simulink model "BC"  (R2019b)
settings: Solver=FixedStepDiscrete  StartTime=0.0  StopTime=stop_time  RelTol=1e-3
InitFcn:
  | sm_callback_init
StopFcn:
  | sm_callback_stop
values from neighbouring files (symbols this model uses):
  mp = sm_init_avalon_signals(mp)    [sm_callback_init.m]
libraries: simulink x5
settings Model: Creator=Ross  LastModifiedBy=bugsbunny
settings DataIOCC: ReturnWorkspaceOutputs=off
settings OptimizationCC: BlockReduction=off  ConditionallyExecuteInputs=off  DefaultParameterBehavior=Inlined
settings DebuggingCC: ReadBeforeWriteMsg=DisableAll  WriteAfterWriteMsg=DisableAll  WriteAfterReadMsg=DisableAll  AlgebraicLoopMsg=error  MultiTaskDSMMsg=none  SingleTaskRateTransMsg=error  PregeneratedLibrarySubsystemCodeDiagnostic=none  ArithmeticOperatorsInVariantConditions=warning
settings HardwareCC: ProdBitPerPointer=32  ProdBitPerSizeT=32  ProdBitPerPtrDiffT=32  ProdLargestAtomicFloat=None  ProdIntDivRoundTo=Undefined  ProdEndianess=Unspecified  ProdWordSize=32  ProdHWDeviceType=ASIC/FPGA->ASIC/FPGA  TargetBitPerPointer=64  TargetBitPerSizeT=64  TargetBitPerPtrDiffT=64  TargetLongLongMode=on  TargetIntDivRoundTo=Zero  TargetEndianess=LittleEndian  TargetWordSize=64  TargetHWDeviceType=Custom Processor->MATLAB Host Computer  ProdEqTarget=off
settings ModelReferenceCC: UpdateModelReferenceTargets=IfOutOfDate
settings SFSimCC: SFSimEcho=off  SimUseLocalCustomCode=off  CustomCodeUndefinedFunction=UseInterfaceOnly
settings RTWCC: RTWUseLocalCustomCode=off

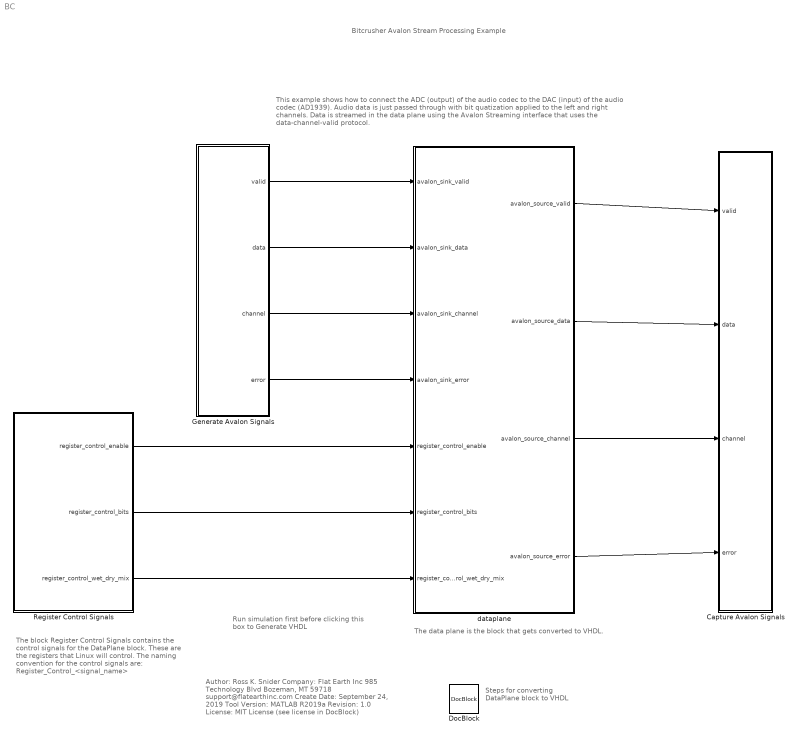
== system BC ==
  note: The data plane is the block that gets converted to VHDL.
  note: Author:          Ross K. Snider
      | Company:     Flat Earth Inc
      |                       985 Technology Blvd
      |                       Bozeman, MT 59718
      |                       support@flatearthinc.com
      | Create Date:  September 24, 2019
      | Tool Version:  MATLAB R2019a
      | Revision:        1.0
      | License:          MIT License (see license in DocBlock)
  note: This example shows how to connect the ADC (output) of the audio codec to the DAC (input) of the audio codec (AD1939). Audio data is just passed through with bit quatization applied to the left and right channels. Data is streamed in the data plane using the Avalon Streaming interface that uses the data-channel-valid protocol.
  note: Steps for converting
      | DataPlane block
      | to VHDL
  note: Bitcrusher
      | Avalon Stream Processing Example
  note: Run simulation first
      | before clicking this box to
      | Generate VHDL
  note: The block Register Control Signals contains
      | the control signals for the DataPlane block.
      | These are the registers that Linux will control.
      | The naming convention for the control
      | signals are:  Register_Control_<signal_name>
  Capture Avalon Signals : Subsystem
  DocBlock : simulink/Model-Wide Utilities/DocBlock  DocumentType=HTML
  Generate Avalon Signals : Subsystem
  Register Control Signals : Subsystem
  dataplane : Subsystem  TreatAsAtomicUnit=on
  wires:
  Generate Avalon Signals/2(data) -> dataplane/2(avalon_sink_data)
  Generate Avalon Signals/1(valid) -> dataplane/1(avalon_sink_valid)
  Generate Avalon Signals/3(channel) -> dataplane/3(avalon_sink_channel)
  Generate Avalon Signals/4(error) -> dataplane/4(avalon_sink_error)
  dataplane/2(avalon_source_data) -> Capture Avalon Signals/2(data)
  dataplane/1(avalon_source_valid) -> Capture Avalon Signals/1(valid)
  dataplane/3(avalon_source_channel) -> Capture Avalon Signals/3(channel)
  dataplane/4(avalon_source_error) -> Capture Avalon Signals/4(error)
  Register Control Signals/2(register_control_bits) -> dataplane/6(register_control_bits)
  Register Control Signals/1(register_control_enable) -> dataplane/5(register_control_enable)
  Register Control Signals/3(register_control_wet_dry_mix) -> dataplane/7(register_control_wet_dry_mix)

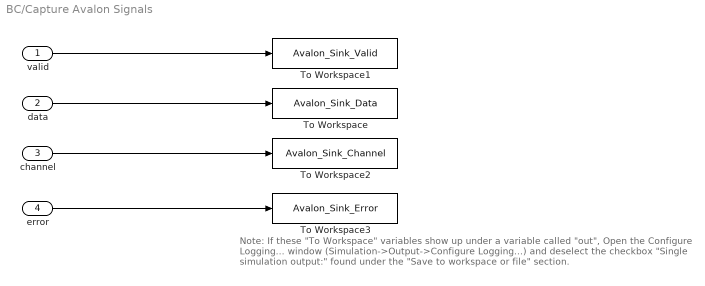
== system BC/Capture Avalon Signals ==
  note: Note:  If these "To Workspace" variables show up under a variable called "out",
      | Open the Configure Logging... window (Simulation->Output->Configure Logging...)
      | and deselect the checkbox "Single simulation output:" found under the "Save to workspace or file" section.
  valid : Inport
  data : Inport  Port=2
  channel : Inport  Port=3
  error : Inport  Port=4
  To Workspace : ToWorkspace  VariableName=Avalon_Sink_Data  SaveFormat=Timeseries  SampleTime=-1
  To Workspace1 : ToWorkspace  VariableName=Avalon_Sink_Valid  SaveFormat=Timeseries  SampleTime=-1
  To Workspace2 : ToWorkspace  VariableName=Avalon_Sink_Channel  SaveFormat=Timeseries  SampleTime=-1
  To Workspace3 : ToWorkspace  VariableName=Avalon_Sink_Error  SaveFormat=Timeseries  SampleTime=-1
  wires:
  data/1 -> To Workspace/1
  valid/1 -> To Workspace1/1
  error/1 -> To Workspace3/1
  channel/1 -> To Workspace2/1

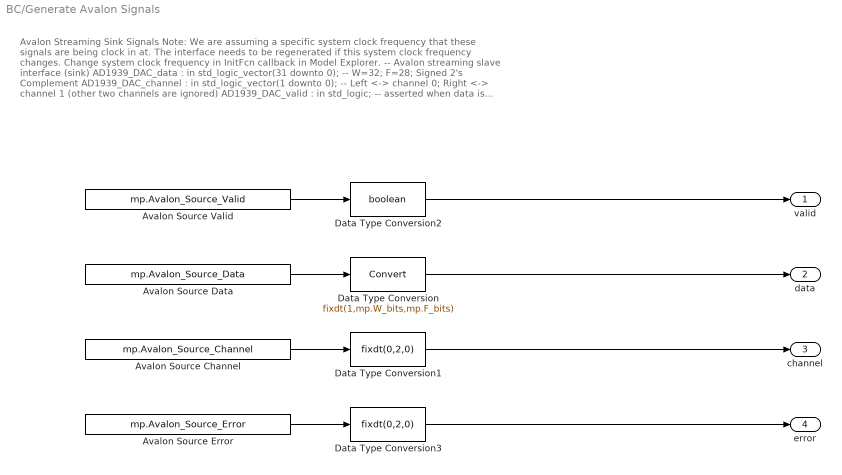
== system BC/Generate Avalon Signals ==
  note: Avalon Streaming Sink Signals
      | Note: We are assuming a specific system clock frequency that these signals are being clock in at.
      | The interface needs to be regenerated if this system clock frequency changes. Change system clock frequency in InitFcn callback in Model Explorer.
      |
      | -- Avalon streaming slave interface (sink)
      | AD1939_DAC_data : in std_logic_vector(31 downto 0); -- W=32; F=28; Signed 2's Complement
      | AD1939_DAC_channel : in std_logic_vector(1 downto 0); -- Left <-> channel 0; Right <-> channel 1 (other two channels are ignored)
      | AD1939_DAC_valid : in std_logic; -- asserted when data is valid
      | AD1939_DAC_error : in std_logic_vector(1 downto 0) -- error channel is ignored, assumed to be error free at this point
      |
      | For more information on the data-channel-valid protocol, s ee chapter 5 in Intel's Avalon Interfaced Specification (p. 40) at https://www.intel.com/content/dam/www/programmable/us/en/pdfs/literature/manual/mnl_avalon_spec.pdf
  Avalon Source Channel : FromWorkspace  VariableName=mp.Avalon_Source_Channel  OutDataTypeStr=double  SampleTime=mp.Ts_system
  "Avalon Source Data " : FromWorkspace  VariableName=mp.Avalon_Source_Data  OutDataTypeStr=double  SampleTime=mp.Ts_system
  Avalon Source Error : FromWorkspace  VariableName=mp.Avalon_Source_Error  OutDataTypeStr=double  SampleTime=mp.Ts_system
  Avalon Source Valid : FromWorkspace  VariableName=mp.Avalon_Source_Valid  OutDataTypeStr=double  SampleTime=mp.Ts_system
  Data Type Conversion : DataTypeConversion  OutDataTypeStr=fixdt(1,mp.W_bits,mp.F_bits)
  Data Type Conversion1 : DataTypeConversion  OutDataTypeStr=fixdt(0,2,0)
  Data Type Conversion2 : DataTypeConversion  OutDataTypeStr=boolean
  Data Type Conversion3 : DataTypeConversion  OutDataTypeStr=fixdt(0,2,0)
  valid : Outport  VectorParamsAs1DForOutWhenUnconnected=off
  data : Outport  Port=2  VectorParamsAs1DForOutWhenUnconnected=off
  channel : Outport  Port=3  VectorParamsAs1DForOutWhenUnconnected=off
  error : Outport  Port=4  VectorParamsAs1DForOutWhenUnconnected=off
  wires:
  Data Type Conversion1/1 -> channel/1
  Data Type Conversion2/1 -> valid/1
  Avalon Source Error/1 -> Data Type Conversion3/1
  Data Type Conversion/1 -> data/1
  Avalon Source Valid/1 -> Data Type Conversion2/1
  Data Type Conversion3/1 -> error/1
  Avalon Source Channel/1 -> Data Type Conversion1/1
  "Avalon Source Data "/1 -> Data Type Conversion/1

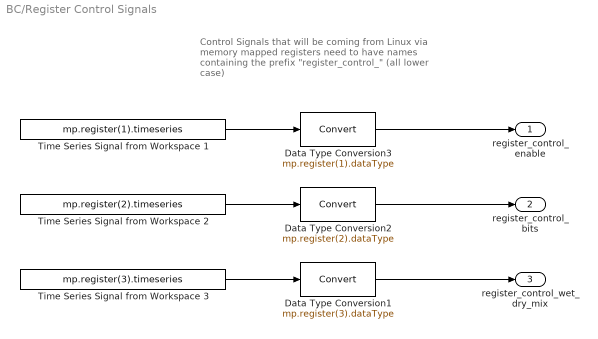
== system BC/Register Control Signals ==
  note: Control Signals that will be coming from Linux via
      | memory mapped registers need to have names
      | containing the prefix "register_control_"
      | (all lower case)
  Data Type Conversion1 : DataTypeConversion  OutDataTypeStr=mp.register(3).dataType
  Data Type Conversion2 : DataTypeConversion  OutDataTypeStr=mp.register(2).dataType
  Data Type Conversion3 : DataTypeConversion  OutDataTypeStr=mp.register(1).dataType
  Time Series Signal from Workspace 1 : FromWorkspace  VariableName=mp.register(1).timeseries  OutDataTypeStr=double  SampleTime=mp.Ts_system
  Time Series Signal from Workspace 2 : FromWorkspace  VariableName=mp.register(2).timeseries  OutDataTypeStr=double  SampleTime=mp.Ts_system
  Time Series Signal from Workspace 3 : FromWorkspace  VariableName=mp.register(3).timeseries  OutDataTypeStr=double  SampleTime=mp.Ts_system
  register_control_enable : Outport  VectorParamsAs1DForOutWhenUnconnected=off
  register_control_bits : Outport  Port=2  VectorParamsAs1DForOutWhenUnconnected=off
  register_control_wet_dry_mix : Outport  Port=3  VectorParamsAs1DForOutWhenUnconnected=off
  wires:
  Time Series Signal from Workspace 2/1 -> Data Type Conversion2/1
  Data Type Conversion2/1 -> register_control_bits/1
  Time Series Signal from Workspace 1/1 -> Data Type Conversion3/1
  Data Type Conversion3/1 -> register_control_enable/1
  Time Series Signal from Workspace 3/1 -> Data Type Conversion1/1
  Data Type Conversion1/1 -> register_control_wet_dry_mix/1

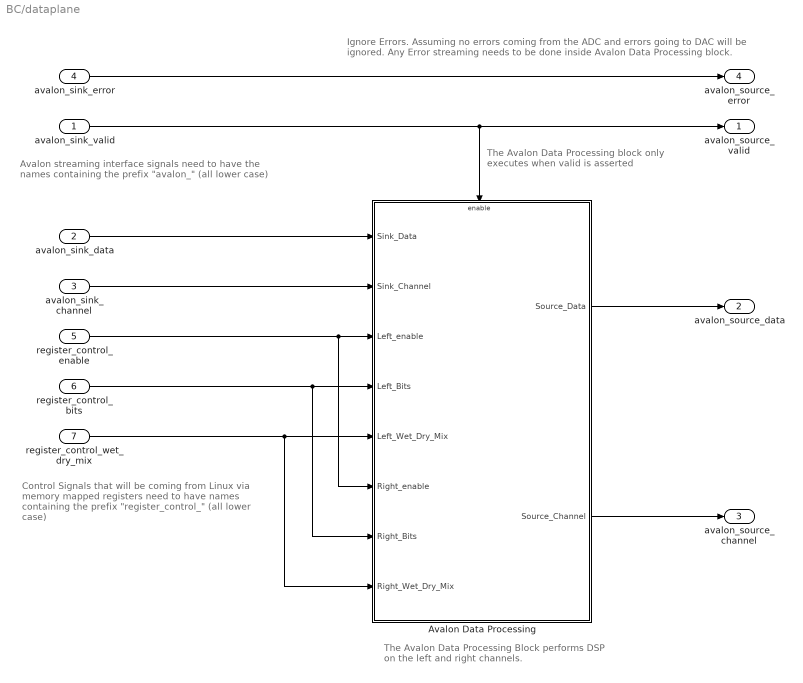
== system BC/dataplane ==
  note: Control Signals that will be coming from Linux via
      | memory mapped registers need to have names
      | containing the prefix "register_control_"
      | (all lower case)
  note: The Avalon Data Processing Block
      | performs DSP on the left and right channels.
  note: The Avalon Data Processing block
      | only executes when valid is asserted
  note: Ignore Errors.
      | Assuming no errors coming from the ADC and errors going to DAC will be ignored.
      | Any Error streaming needs to be done inside Avalon Data Processing block.
  note: Avalon streaming interface signals need to have the
      | names containing the prefix "avalon_"
      | (all lower case)
  avalon_sink_valid : Inport
  avalon_sink_data : Inport  Port=2
  avalon_sink_channel : Inport  Port=3
  avalon_sink_error : Inport  Port=4
  register_control_enable : Inport  Port=5
  register_control_bits : Inport  Port=6
  register_control_wet_dry_mix : Inport  Port=7
  Avalon Data Processing : Subsystem  TreatAsAtomicUnit=on
  avalon_source_valid : Outport  VectorParamsAs1DForOutWhenUnconnected=off
  avalon_source_data : Outport  Port=2  VectorParamsAs1DForOutWhenUnconnected=off
  avalon_source_channel : Outport  Port=3  VectorParamsAs1DForOutWhenUnconnected=off
  avalon_source_error : Outport  Port=4  VectorParamsAs1DForOutWhenUnconnected=off
  wires:
  avalon_sink_channel/1 -> Avalon Data Processing/2(Sink_Channel)
  avalon_sink_error/1 -> avalon_source_error/1
  Avalon Data Processing/1(Source_Data) -> avalon_source_data/1
  avalon_sink_valid/1 -> avalon_source_valid/1, Avalon Data Processing/Enable
  avalon_sink_data/1 -> Avalon Data Processing/1(Sink_Data)
  Avalon Data Processing/2(Source_Channel) -> avalon_source_channel/1
  register_control_bits/1 -> Avalon Data Processing/7(Right_Bits), Avalon Data Processing/4(Left_Bits)
  register_control_enable/1 -> Avalon Data Processing/6(Right_enable), Avalon Data Processing/3(Left_enable)
  register_control_wet_dry_mix/1 -> Avalon Data Processing/8(Right_Wet_Dry_Mix), Avalon Data Processing/5(Left_Wet_Dry_Mix)

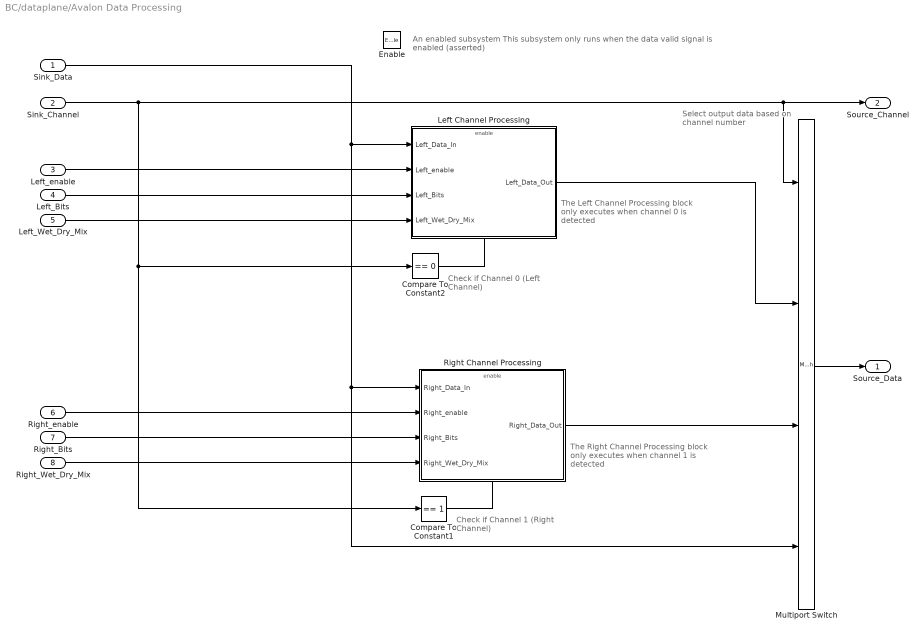
== system BC/dataplane/Avalon Data Processing ==
  note: Select output data
      | based on channel number
  note: Check if Channel 0
      | (Left Channel)
  note: The Left Channel Processing block
      | only executes when channel 0
      | is detected
  note: The Right Channel Processing block
      | only executes when channel 1
      | is detected
  note: Check if Channel 1
      | (Right Channel)
  note: An enabled subsystem
      | This subsystem only runs when the data valid signal is enabled (asserted)
  Sink_Data : Inport
  Sink_Channel : Inport  Port=2
  Left_enable : Inport  Port=3
  Left_Bits : Inport  Port=4
  Left_Wet_Dry_Mix : Inport  Port=5
  Right_enable : Inport  Port=6
  Right_Bits : Inport  Port=7
  Right_Wet_Dry_Mix : Inport  Port=8
  Enable : EnablePort
  Compare To Constant1 : simulink/Logic and Bit Operations/Compare To Constant  relop===  const=1  OutDataTypeStr=boolean
  Compare To Constant2 : simulink/Logic and Bit Operations/Compare To Constant  relop===  const=0  OutDataTypeStr=boolean
  Left Channel Processing : Subsystem  TreatAsAtomicUnit=on
  Multiport Switch : MultiPortSwitch  DataPortOrder=Zero-based contiguous  zeroidx=on
  Right Channel Processing : Subsystem  TreatAsAtomicUnit=on
  Source_Data : Outport  InitialOutput=0  VectorParamsAs1DForOutWhenUnconnected=off
  Source_Channel : Outport  Port=2  InitialOutput=0  VectorParamsAs1DForOutWhenUnconnected=off
  wires:
  Sink_Channel/1 -> Compare To Constant1/1, Compare To Constant2/1, Source_Channel/1, Multiport Switch/1
  Compare To Constant2/1 -> Left Channel Processing/Enable
  Compare To Constant1/1 -> Right Channel Processing/Enable
  Sink_Data/1 -> Multiport Switch/4, Right Channel Processing/1(Right_Data_In), Left Channel Processing/1(Left_Data_In)
  Left Channel Processing/1("Left_Data_Out ") -> Multiport Switch/2
  Right Channel Processing/1("Right_Data_Out ") -> Multiport Switch/3
  Multiport Switch/1 -> Source_Data/1
  Left_Bits/1 -> Left Channel Processing/3(Left_Bits)
  Right_Bits/1 -> Right Channel Processing/3(Right_Bits)
  Left_enable/1 -> Left Channel Processing/2(Left_enable)
  Right_enable/1 -> Right Channel Processing/2(Right_enable)
  Left_Wet_Dry_Mix/1 -> Left Channel Processing/4(Left_Wet_Dry_Mix)
  Right_Wet_Dry_Mix/1 -> Right Channel Processing/4(Right_Wet_Dry_Mix)

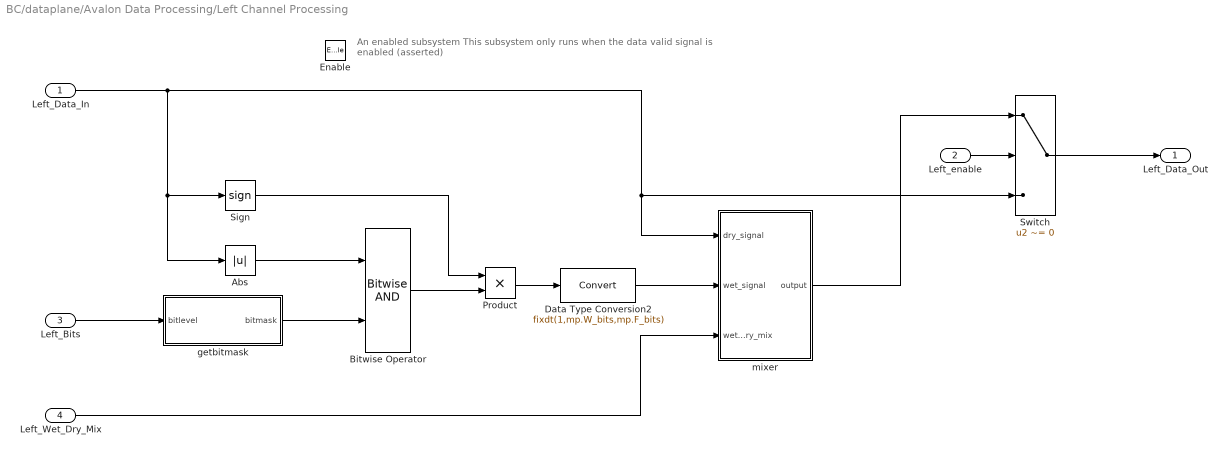
== system BC/dataplane/Avalon Data Processing/Left Channel Processing ==
  note: An enabled subsystem
      | This subsystem only runs when the data valid signal is enabled (asserted)
  Left_Data_In : Inport
  Left_enable : Inport  Port=2
  Left_Bits : Inport  Port=3
  Left_Wet_Dry_Mix : Inport  Port=4
  Enable : EnablePort
  Abs : Abs  OutDataTypeStr=fixdt(0,32,28)
  Bitwise Operator : simulink/Logic and Bit Operations/Bitwise Operator  logicop=AND  UseBitMask=off  NumInputPorts=2  BitMask=bin2dec('11011001')  BitMaskRealWorld=Stored Integer
  Data Type Conversion2 : DataTypeConversion  OutDataTypeStr=fixdt(1,mp.W_bits,mp.F_bits)
  Product : Product
  Sign : Signum
  Switch : Switch  Criteria=u2 ~= 0
  getbitmask : MATLAB Function  TreatAsAtomicUnit=on
  mixer : Subsystem
  "Left_Data_Out " : Outport  InitialOutput=0  VectorParamsAs1DForOutWhenUnconnected=off
  wires:
  Left_Bits/1 -> getbitmask/1(bitlevel)
  getbitmask/1(bitmask) -> Bitwise Operator/2
  Left_Data_In/1 -> Abs/1, Sign/1, mixer/1(dry_signal), Switch/3
  Abs/1 -> Bitwise Operator/1
  Product/1 -> Data Type Conversion2/1
  Bitwise Operator/1 -> Product/2
  Sign/1 -> Product/1
  Switch/1 -> "Left_Data_Out "/1
  Data Type Conversion2/1 -> mixer/2(wet_signal)
  Left_Wet_Dry_Mix/1 -> mixer/3(wet_dry_mix)
  Left_enable/1 -> Switch/2
  mixer/1(output) -> Switch/1

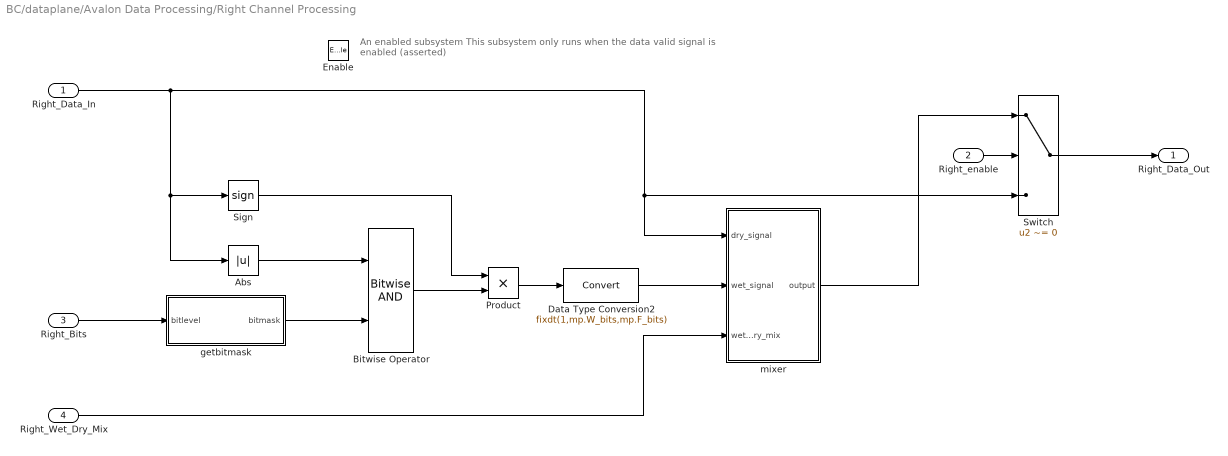
== system BC/dataplane/Avalon Data Processing/Right Channel Processing ==
  note: An enabled subsystem
      | This subsystem only runs when the data valid signal is enabled (asserted)
  Right_Data_In : Inport
  Right_enable : Inport  Port=2
  Right_Bits : Inport  Port=3
  Right_Wet_Dry_Mix : Inport  Port=4
  Enable : EnablePort
  Abs : Abs  OutDataTypeStr=fixdt(0,32,28)
  Bitwise Operator : simulink/Logic and Bit Operations/Bitwise Operator  logicop=AND  UseBitMask=off  NumInputPorts=2  BitMask=bin2dec('11011001')  BitMaskRealWorld=Stored Integer
  Data Type Conversion2 : DataTypeConversion  OutDataTypeStr=fixdt(1,mp.W_bits,mp.F_bits)
  Product : Product
  Sign : Signum
  Switch : Switch  Criteria=u2 ~= 0
  getbitmask : MATLAB Function  TreatAsAtomicUnit=on
  mixer : Subsystem
  "Right_Data_Out " : Outport  InitialOutput=0  VectorParamsAs1DForOutWhenUnconnected=off
  wires:
  Right_Bits/1 -> getbitmask/1(bitlevel)
  getbitmask/1(bitmask) -> Bitwise Operator/2
  Right_Data_In/1 -> Abs/1, Sign/1, Switch/3, mixer/1(dry_signal)
  Abs/1 -> Bitwise Operator/1
  Product/1 -> Data Type Conversion2/1
  Bitwise Operator/1 -> Product/2
  Sign/1 -> Product/1
  Switch/1 -> "Right_Data_Out "/1
  Data Type Conversion2/1 -> mixer/2(wet_signal)
  Right_Wet_Dry_Mix/1 -> mixer/3(wet_dry_mix)
  mixer/1(output) -> Switch/1
  Right_enable/1 -> Switch/2

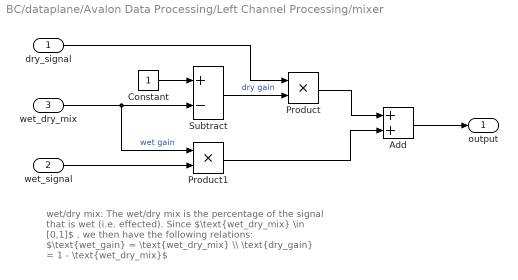
== system BC/dataplane/Avalon Data Processing/Left Channel Processing/mixer ==
  note: wet/dry mix:
      | The wet/dry mix is the percentage of the signal that is wet (i.e. effected).
      |
      | Since $\text{wet_dry_mix} \in [0,1]$ , we then have the following relations:
      | $\text{wet_gain} = \text{wet_dry_mix} \\ \text{dry_gain} = 1 - \text{wet_dry_mix}$
  dry_signal : Inport
  wet_signal : Inport  Port=2
  wet_dry_mix : Inport  Port=3
  Add : Sum  OutDataTypeStr=fixdt(1,mp.W_bits,mp.F_bits)
  Constant : Constant  OutDataTypeStr=Inherit: Inherit via back propagation  SampleTime=-1
  Product : Product  OutDataTypeStr=Inherit: Keep MSB
  Product1 : Product  OutDataTypeStr=Inherit: Keep MSB
  Subtract : Sum  Inputs=+-  InputSameDT=on  OutDataTypeStr=Inherit: Same as first input
  output : Outport  VectorParamsAs1DForOutWhenUnconnected=off
  wires:
  Add/1 -> output/1
  Constant/1 -> Subtract/1
  wet_dry_mix/1 -> Product1/1, Subtract/2  "wet gain"
  Product/1 -> Add/1
  Product1/1 -> Add/2
  wet_signal/1 -> Product1/2
  dry_signal/1 -> Product/1
  Subtract/1 -> Product/2  "dry gain"

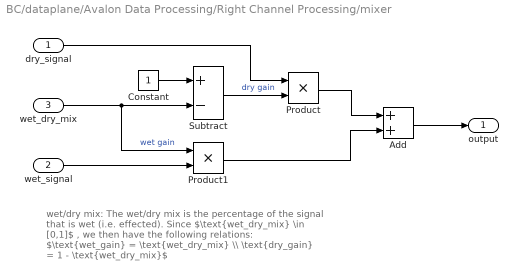
== system BC/dataplane/Avalon Data Processing/Right Channel Processing/mixer ==
  note: wet/dry mix:
      | The wet/dry mix is the percentage of the signal that is wet (i.e. effected).
      |
      | Since $\text{wet_dry_mix} \in [0,1]$ , we then have the following relations:
      | $\text{wet_gain} = \text{wet_dry_mix} \\ \text{dry_gain} = 1 - \text{wet_dry_mix}$
  dry_signal : Inport
  wet_signal : Inport  Port=2
  wet_dry_mix : Inport  Port=3
  Add : Sum  OutDataTypeStr=fixdt(1,mp.W_bits,mp.F_bits)
  Constant : Constant  OutDataTypeStr=Inherit: Inherit via back propagation  SampleTime=-1
  Product : Product  OutDataTypeStr=Inherit: Keep MSB
  Product1 : Product  OutDataTypeStr=Inherit: Keep MSB
  Subtract : Sum  Inputs=+-  InputSameDT=on  OutDataTypeStr=Inherit: Same as first input
  output : Outport  VectorParamsAs1DForOutWhenUnconnected=off
  wires:
  Product1/1 -> Add/2
  Product/1 -> Add/1
  dry_signal/1 -> Product/1
  Subtract/1 -> Product/2  "dry gain"
  wet_dry_mix/1 -> Product1/1, Subtract/2  "wet gain"
  Constant/1 -> Subtract/1
  Add/1 -> output/1
  wet_signal/1 -> Product1/2

== matlab function BC/dataplane/Avalon Data Processing/Right Channel Processing/getbitmask ==
  data: bitlevel input; bitmask output
function bitmask = getbitmask(bitlevel)
bitmask=fi(0,0,32,28);
switch(bitlevel)
    case 0
        bitmask = fi(0.0000000000000000000000000000,0,32,28);
    case 1
        bitmask = fi(8.0000000000000000000000000000,0,32,28);
    case 2
        bitmask = fi(12.0000000000000000000000000000,0,32,28);
    case 3
        bitmask = fi(14.0000000000000000000000000000,0,32,28);
    case 4
        bitmask = fi(15.0000000000000000000000000000,0,32,28);
    case 5
        bitmask = fi(15.5000000000000000000000000000,0,32,28);
    case 6
        bitmask = fi(15.7500000000000000000000000000,0,32,28);
    case 7
        bitmask = fi(15.8750000000000000000000000000,0,32,28);
    case 8
        bitmask = fi(15.9375000000000000000000000000,0,32,28);
    case 9
        bitmask = fi(15.9687500000000000000000000000,0,32,28);
    case 10
        bitmask = fi(15.9843750000000000000000000000,0,32,28);
    case 11
        bitmask = fi(15.9921875000000000000000000000,0,32,28);
    case 12
        bitmask = fi(15.9960937500000000000000000000,0,32,28);
    case 13
        bitmask = fi(15.9980468750000000000000000000,0,32,28);
    case 14
        bitmask = fi(15.9990234375000000000000000000,0,32,28);
    case 15
        bitmask = fi(15.9995117187500000000000000000,0,32,28);
    case 16
        bitmask = fi(15.9997558593750000000000000000,0,32,28);
    case 17
        bitmask = fi(15.9998779296875000000000000000,0,32,28);
    case 18
        bitmask = fi(15.9999389648437500000000000000,0,32,28);
    case 19
        bitmask = fi(15.9999694824218750000000000000,0,32,28);
    case 20
        bitmask = fi(15.9999847412109375000000000000,0,32,28);
    case 21
        bitmask = fi(15.9999923706054687500000000000,0,32,28);
    case 22
        bitmask = fi(15.9999961853027343750000000000,0,32,28);
    case 23
        bitmask = fi(15.9999980926513671875000000000,0,32,28);
    case 24
        bitmask = fi(15.9999990463256835937500000000,0,32,28);
    case 25
        bitmask = fi(15.9999995231628417968750000000,0,32,28);
    case 26
        bitmask = fi(15.9999997615814208984375000000,0,32,28);
    case 27
        bitmask = fi(15.9999998807907104492187500000,0,32,28);
    case 28
        bitmask = fi(15.9999999403953552246093750000,0,32,28);
    case 29
        bitmask = fi(15.9999999701976776123046875000,0,32,28);
    case 30
        bitmask = fi(15.9999999850988388061523437500,0,32,28);
    case 31
        bitmask = fi(15.9999999925494194030761718750,0,32,28);
    case 32
        bitmask = fi(15.9999999962747097015380859375,0,32,28);
end

== matlab function BC/dataplane/Avalon Data Processing/Left Channel Processing/getbitmask ==
  data: bitlevel input; bitmask output
function bitmask = getbitmask(bitlevel)
bitmask=fi(0,0,32,28);
switch(bitlevel)
    case 0
        bitmask = fi(0.0000000000000000000000000000,0,32,28);
    case 1
        bitmask = fi(8.0000000000000000000000000000,0,32,28);
    case 2
        bitmask = fi(12.0000000000000000000000000000,0,32,28);
    case 3
        bitmask = fi(14.0000000000000000000000000000,0,32,28);
    case 4
        bitmask = fi(15.0000000000000000000000000000,0,32,28);
    case 5
        bitmask = fi(15.5000000000000000000000000000,0,32,28);
    case 6
        bitmask = fi(15.7500000000000000000000000000,0,32,28);
    case 7
        bitmask = fi(15.8750000000000000000000000000,0,32,28);
    case 8
        bitmask = fi(15.9375000000000000000000000000,0,32,28);
    case 9
        bitmask = fi(15.9687500000000000000000000000,0,32,28);
    case 10
        bitmask = fi(15.9843750000000000000000000000,0,32,28);
    case 11
        bitmask = fi(15.9921875000000000000000000000,0,32,28);
    case 12
        bitmask = fi(15.9960937500000000000000000000,0,32,28);
    case 13
        bitmask = fi(15.9980468750000000000000000000,0,32,28);
    case 14
        bitmask = fi(15.9990234375000000000000000000,0,32,28);
    case 15
        bitmask = fi(15.9995117187500000000000000000,0,32,28);
    case 16
        bitmask = fi(15.9997558593750000000000000000,0,32,28);
    case 17
        bitmask = fi(15.9998779296875000000000000000,0,32,28);
    case 18
        bitmask = fi(15.9999389648437500000000000000,0,32,28);
    case 19
        bitmask = fi(15.9999694824218750000000000000,0,32,28);
    case 20
        bitmask = fi(15.9999847412109375000000000000,0,32,28);
    case 21
        bitmask = fi(15.9999923706054687500000000000,0,32,28);
    case 22
        bitmask = fi(15.9999961853027343750000000000,0,32,28);
    case 23
        bitmask = fi(15.9999980926513671875000000000,0,32,28);
    case 24
        bitmask = fi(15.9999990463256835937500000000,0,32,28);
    case 25
        bitmask = fi(15.9999995231628417968750000000,0,32,28);
    case 26
        bitmask = fi(15.9999997615814208984375000000,0,32,28);
    case 27
        bitmask = fi(15.9999998807907104492187500000,0,32,28);
    case 28
        bitmask = fi(15.9999999403953552246093750000,0,32,28);
    case 29
        bitmask = fi(15.9999999701976776123046875000,0,32,28);
    case 30
        bitmask = fi(15.9999999850988388061523437500,0,32,28);
    case 31
        bitmask = fi(15.9999999925494194030761718750,0,32,28);
    case 32
        bitmask = fi(15.9999999962747097015380859375,0,32,28);
end
